simulink model "LedRGB"  (R2017a)
settings: Solver=FixedStepAuto  StartTime=0.0  StopTime=inf  FixedStep=0.01  RelTol=1e-3
PostLoadFcn:
  | try
  |   open(UI_LedRGB)
  | end
libraries: arduinolib x3, simulink x3
CloseFcn:
  | try
  |   close(UI_LedRGB)
  | end
settings Model: SimulationMode=external  ExtModeTrigDuration=2  Creator=ocommeng  LastModifiedBy=ocommeng
settings OptimizationCC: PassReuseOutputArgsAs=Individual arguments  MaxStackSize=64
settings DebuggingCC: ParameterTunabilityLossMsg=error
settings HardwareCC: ProdBitPerInt=16  ProdBitPerPointer=16  ProdBitPerSizeT=16  ProdBitPerPtrDiffT=16  ProdLargestAtomicFloat=None  ProdWordSize=8  ProdHWDeviceType=Atmel->AVR
settings SFSimCC: MATLABDynamicMemAlloc=off
settings RTWCC: SystemTargetFile=ert.tlc  HardwareBoard=Arduino Uno  TLCOptions=-aInlineSetEventsForThisBaseRateFcn=TLC_FALSE -aSuppressMultiTaskScheduler=TLC_FALSE -aRateBasedStepFcn=1  TemplateMakefile=ert_default_tmf  Description=Embedded Coder  GenerateReport=on  Toolchain=Arduino AVR  BuildConfiguration=Faster Runs  IncludeHyperlinkInReport=on  LaunchReport=on  GenerateTraceInfo=on  GenerateTraceReport=on  GenerateTraceReportSl=on  GenerateTraceReportSf=on  GenerateTraceReportEml=on
settings CodeAppCC: ForceParamTrailComments=on  IgnoreCustomStorageClasses=off  OperatorAnnotations=on  SimulinkDataObjDesc=on  SFDataObjDesc=on  MATLABFcnDesc=on  InsertBlockDesc=on  MATLABSourceComments=on
settings ERTTargetCC: SupportContinuousTime=on  SupportVariableSizeSignals=on

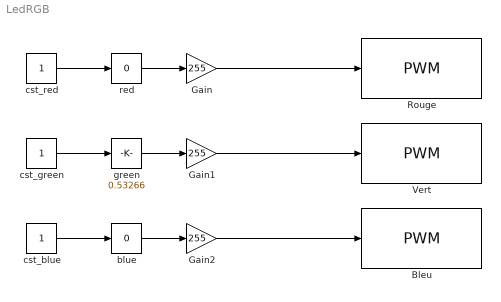
== system LedRGB ==
  "Bleu " : arduinolib/PWM  pinNumber=11  blockPlatform=arduino
  Gain : Gain  Gain=255
  Gain1 : Gain  Gain=255
  Gain2 : Gain  Gain=255
  Rouge : arduinolib/PWM  pinNumber=9  blockPlatform=arduino
  Vert : arduinolib/PWM  pinNumber=10  blockPlatform=arduino
  blue : simulink/Math Operations/Slider Gain  gain=0  low=0  high=1
      settings: AttributesFormatString=%<gain>
  cst_blue : Constant
  "cst_green " : Constant
  cst_red : Constant
  green : simulink/Math Operations/Slider Gain  gain=0.53266  low=0  high=1
  red : simulink/Math Operations/Slider Gain  gain=0  low=0  high=1
  wires:
  cst_red/1 -> red/1
  "cst_green "/1 -> green/1
  cst_blue/1 -> blue/1
  Gain/1 -> Rouge/1
  Gain1/1 -> Vert/1
  Gain2/1 -> "Bleu "/1
  red/1 -> Gain/1
  green/1 -> Gain1/1
  blue/1 -> Gain2/1
